simulink model "lista2_item_j"  (R2014b)
settings: Solver=ode45  StartTime=0.0  StopTime=Tsim  RelTol=1e-3
values from neighbouring files (symbols this model uses):
  T = 1    [sistema_lista3.m]
libraries: cstblocks x5
settings Model: Creator=Danilo  LastModifiedBy=Danilo

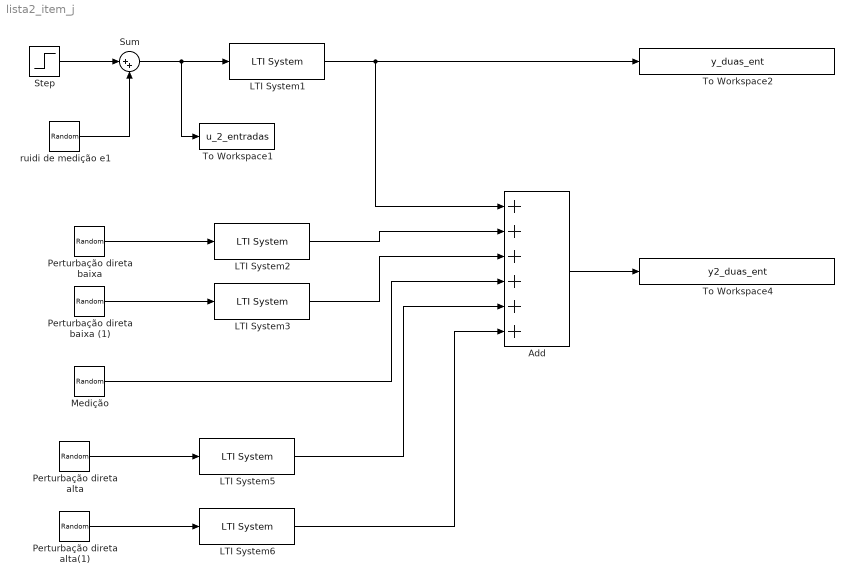
== system lista2_item_j ==
  Add : Sum  Inputs=++++++
  LTI System1 : cstblocks/LTI System  sys=H  IC=[]
  LTI System2 : cstblocks/LTI System  sys=G_pert_1  IC=[]
  LTI System3 : cstblocks/LTI System  sys=G_pert_2  IC=[]
  LTI System5 : cstblocks/LTI System  sys=G_pert_1  IC=[]
  LTI System6 : cstblocks/LTI System  sys=G_pert_2  IC=[]
  Medição : RandomNumber  Variance=exp(-6)  Seed=24  SampleTime=0.1
  Perturbação direta alta : RandomNumber  Variance=0.1  Seed=99  SampleTime=0.1
  Perturbação direta alta(1) : RandomNumber  Variance=0.1  Seed=22  SampleTime=0.1
  Perturbação direta baixa : RandomNumber  Variance=0.001  SampleTime=0.1
  Perturbação direta baixa (1) : RandomNumber  Variance=0.001  Seed=12  SampleTime=0.1
  Step : Step  Time=0  Before=0.1  After=0.1  SampleTime=1
  Sum : Sum  Inputs=|++
  To Workspace1 : ToWorkspace  VariableName=u_2_entradas  SampleTime=T
  To Workspace2 : ToWorkspace  VariableName=y_duas_ent  SampleTime=T
  To Workspace4 : ToWorkspace  VariableName=y2_duas_ent  SampleTime=T
  "ruidi de medição e1 " : RandomNumber  Variance=exp(-6)  SampleTime=0.1
  wires:
  LTI System1/1 -> Add/1, To Workspace2/1
  Add/1 -> To Workspace4/1
  Perturbação direta baixa/1 -> LTI System2/1
  Perturbação direta baixa (1)/1 -> LTI System3/1
  LTI System2/1 -> Add/2
  LTI System3/1 -> Add/3
  Medição/1 -> Add/4
  Perturbação direta alta/1 -> LTI System5/1
  Perturbação direta alta(1)/1 -> LTI System6/1
  LTI System5/1 -> Add/5
  LTI System6/1 -> Add/6
  Step/1 -> Sum/1
  "ruidi de medição e1 "/1 -> Sum/2
  Sum/1 -> To Workspace1/1, LTI System1/1
